simulink model "transfig_diagram"  (R2024b)
settings: Solver=VariableStepAuto  StartTime=0.0  StopTime=10.0  RelTol=1e-3
settings Model: Creator=uig58267  LastModifiedBy=Stefania
settings DebuggingCC: SignalResolutionControl=TryResolveAllWithWarning  UnconnectedInputMsg=warning  UnconnectedOutputMsg=warning  UnconnectedLineMsg=warning
settings ModelReferenceCC: EnableRefExpFcnMdlSchedulingChecks=on
settings RTWCC: GPUComputeCapability=3.5  DLArmComputeVersion=19.05

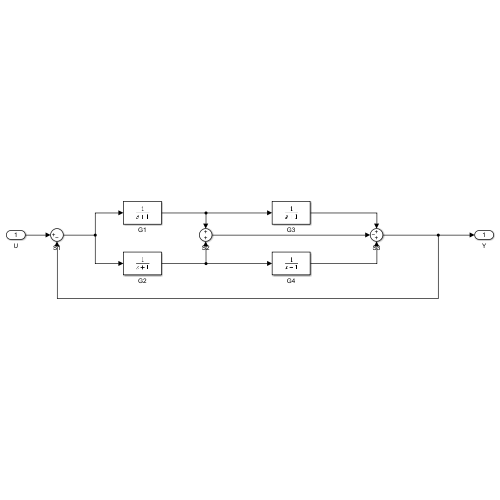
[thumbnail: Simulink's stored preview of the top-level diagram]
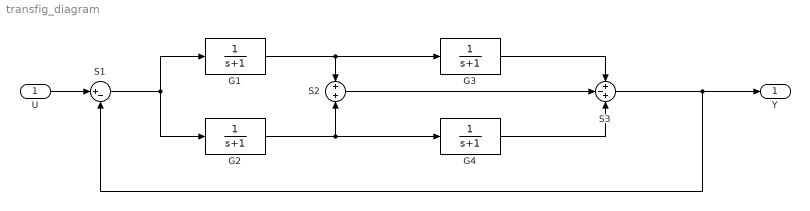
== system transfig_diagram ==
  U : Inport
  G{1..4} (4 alike) : TransferFcn  Denominator=[1 1]
  S1 : Sum  Inputs=|+-
  S2 : Sum
  S3 : Sum  Inputs=+-+
  Y : Outport
  wires:
  U/1 -> S1/1
  S1/1 -> G1/1, G2/1
  G1/1 -> G3/1, S2/1
  G2/1 -> G4/1, S2/2
  S2/1 -> S3/2
  G3/1 -> S3/1
  G4/1 -> S3/3
  S3/1 -> S1/2, Y/1
